simulink model "RoboBoat_SLAM_6_29"  (R2014a)
settings: Solver=FixedStepDiscrete  StartTime=0.0  StopTime=inf  FixedStep=.1  RelTol=1e-3
undefined symbols (not defined in the file): Com1, Com2, Com3, Com4, DiscIntNeverNeededParam, standard
libraries: xpcseriallib x29, visiontextngfix x25, simulink x21, slrtlib x7, speedgoatlib_IO102 x5, speedgoatlib x1
(part 2 of 6)

== matlab function RoboBoat_SLAM_6_29/Main FSM/Obstacle Navigation1/Exit Gate/Gate 1 (Red & White)/MATLAB Function ==
  data: Prob input; RPM output; ColorID input; Dist input; Ang input; CurrentHeading input; GPSLat input; GPSLong input; Timer input; DesiredHeading output; gateGPS output
function [RPM,DesiredHeading,gateGPS] = navigation(Prob,ColorID,Dist,Ang,CurrentHeading,GPSLat,GPSLong,Timer)

% Function performs one buoy navigation through the start speed gates. If
% no buoys are found by the LIDAR/Vision assembly then an incremented
% turning algorithm is executed to turn by 10 degrees per increment up to 
% 90 degrees either way of the inital heading

% Written by Edward Zhu

persistent LockHeading TimeLastFound Counter Turn TurnInc gateLat gateLong

if isempty(LockHeading) && isempty(TimeLastFound) && isempty(Counter) && isempty(Turn) && isempty(TurnInc)
    LockHeading = CurrentHeading;
    TimeLastFound = 0;
    Counter = 0;
    TurnInc = 30;
    Turn = TurnInc;
    gateLat = 0;
    gateLong = 0;
end

Distance = Dist/100;

BoatWidth = 0.75;
Buffer = atan(2*BoatWidth/Distance);

RedOffset = Ang + Buffer;
WhiteOffset = Ang - Buffer;

R = 6378137;

CurLat = (floor(GPSLat/100)+mod(GPSLat,100)/60)*pi/180;
CurLong = (ceil(GPSLong/100)-mod(-GPSLong,100)/60)*pi/180;

gateHeading = (mod(CurrentHeading + Ang, 360))*pi/180;

if ColorID == 1 && Prob > 0.9
    if Ang < 0
        DesiredHeading = mod(CurrentHeading - RedOffset, 360);
    else
        DesiredHeading = mod(CurrentHeading + RedOffset, 360);
    end
    RPM = 4000;
    GateFound = 1;
    TimeLastFound = Timer;
    gateLat =  asin(sin(CurLat)*cos(Distance/R) + cos(CurLat)*sin(Distance/R)*cos(gateHeading))*180/pi;
    gateLong = (CurLong + atan2(sin(gateHeading)*sin(Distance/R)*cos(CurLat),cos(Distance/R)-sin(CurLat)*sin(gateLat)))*180/pi;
elseif ColorID == 2 && Prob > 0.9
    DesiredHeading = mod(LockHeading - Turn, 360);
    RPM = 0;
    GateFound = 1;
    TimeLastFound = Timer;
%     DesiredHeading = mod(CurrentHeading - WhiteOffset, 360);
%     RPM = 4000;
%     GateFound = 1;
%     TimeLastFound = Timer;
%     gateLat =  asin(sin(CurLat)*cos(Distance/R) + cos(CurLat)*sin(Distance/R)*cos(gateHeading))*180/pi;
%     gateLong = (CurLong + atan2(sin(gateHeading)*sin(Distance/R)*cos(CurLat),cos(Distance/R)-sin(CurLat)*sin(gateLat)))*180/pi;
else
    DesiredHeading = CurrentHeading;
    RPM = 0;
    GateFound = 0;
end

gateGPS = [gateLat gateLong];
TimeNoBuoys = Timer - TimeLastFound;

if GateFound == 0 && TimeNoBuoys > 15
    RPM = 0;
    DesiredHeading = mod(LockHeading - Turn, 360);
    HeadingDiff = DesiredHeading - CurrentHeading;
    gateGPS = [gateLat gateLong];
    
    if HeadingDiff > 180
        HeadingDiff = HeadingDiff - 360;
    elseif HeadingDiff < -180
        HeadingDiff = HeadingDiff + 360;
    end
    
    if HeadingDiff < 3
        Counter = Counter + 1;
    else
        Counter = 0;
    end
    
    if Counter >= 15
        Turn = Turn + TurnInc;
        Counter = 0;
        if abs(Turn) > 90
            TurnInc = -TurnInc;
        end
    end
end

== matlab function RoboBoat_SLAM_6_29/Main FSM/Start Speed/GPS Enabler ==
  data: Finished input; SSMode output; Gate1 output; Gate2 output
function [SSMode, Gate1, Gate2] = GPSEnable(Finished)

%Written by Anderson Lebbad on June 9, 2015
%Last Edited: June 10, 2015
%
%This function enables Speedgate tasks. First the searches for and
%navigates through one gate, then the second.

%Initialize Enablers
Gate1 = 0;
Gate2 = 0;


%Switches the enable signal based on which task is flagged as done.
if Finished == 0
    Gate1 = 1;
    SSMode = 1;
else
    Gate2 = 1;
    SSMode = 2;
end

== matlab function RoboBoat_SLAM_6_29/Main FSM/Start Speed/Gate Find and Through/Find/MATLAB Function1 ==
  data: Dist input; Angles input; X input; Y input; Heading input; found output; Goal output; DesiredHeading output
function [found, Goal, DesiredHeading] = SpeedGate(Dist,Angles,X,Y,Heading)
%Written by Anderson Lebbad on May 29, 2015
%Last Edited by:

%This function sends theboat forward until a landmark is found, then it
%navigates towards the right of it.

persistent goalX goalY Found initialHeading change
if isempty(goalX)
    goalX = X;
    goalY = Y;
    Found = 0;
    initialHeading = Heading;
    change = 10;
end

DesiredHeading = Heading;
DistM = Dist./100;
dodgeWidth = 3;

if Found == 0
    if DistM(2) ~= 0
        %If two objects are found, set goal between the two
        w = (DistM(1)*sin(Angles(1)) + DistM(2)*sin(Angles(2)*pi/180)) / 2;
        h = (DistM(1)*cos(Angles(1)) + DistM(2)*sin(Angles(2)*pi/180)) / 2;
        goalX = X + h*cos(Heading) - w*sin(Heading);
        goalY = Y + h*sin(Heading) + w*cos(Heading);
        Found = 1;
    elseif DistM(1) ~= 0
        %If one object is found, set goal dodgewidth to the right of it
        w = DistM(1)*sin(Angles(1)) + dodgeWidth;
        h = DistM(1)*cos(Angles(1));
        goalX = X + h*cos(Heading) - w*sin(Heading);
        goalY = Y + h*sin(Heading) + w*cos(Heading);
        Found = 1;
    else
        %If no objects are found, search. Scan 30 degrees to left and right
        %of initial heading.
        DesiredHeading = Heading + change;
        if abs(DesiredHeading - initialHeading) > 30
            change = -change;
            DesiredHeading = Heading + change;
        end
    end
end

Goal = [goalX, goalY];
found = Found;

end

== matlab function RoboBoat_SLAM_6_29/Main FSM/Obstacle Navigation1/Enter Gate/Gate 2 (White & White)/Distance ==
  data: Distance output; DesiredGPS input; GPSLat input; GPSLong input
function Distance  = DistCalc(DesiredGPS, GPSLat, GPSLong)

%Written by Anderson Lebbad on July 22, 2013
%Last Edited:

%Orients the boat towards a target GPS point before approaching it.
%This is done to keep the approach angle minimal, so the approach
%algorithm does not circle the target and never reach it.

%Parse input GPS and convert angles to radians
CurLat = (floor(GPSLat/100)+mod(GPSLat,100)/60)*pi/180;
CurLong = (floor(GPSLong/100)+mod(GPSLong,100)/60)*pi/180;
DesLat = (floor(DesiredGPS(1)/100)+mod(DesiredGPS(1),100)/60)*pi/180;
DesLong = (floor(DesiredGPS(2)/100)+mod(DesiredGPS(2),100)/60)*pi/180;
%Difference between lats and longs
DiffLat = DesLat - CurLat;
MidLat = cos((CurLat + DesLat)/2);
DiffLong = DesLong - CurLong;
%Radius of the earth in meters
R = 6378137;

%Calculate distance using the great-circle distance formula
%Formula documented here:
%   http://www.movable-type.co.uk/scripts/latlong.html
% a = sin(DiffLat/2)^2+sin(DiffLong/2)^2*cos(CurLat)*cos(DesLat);
% c = 2*atan2(sqrt(a), sqrt(1-a));
% Distance = R*c;

%Calculating distance using Pythagora's
a = DiffLong*MidLat;
b = DiffLat;
Distance = R*sqrt(a^2+b^2);

== matlab function RoboBoat_SLAM_6_29/Main FSM/Obstacle Navigation1/Enter Gate/MATLAB Function ==
  data: gateID input; outputSelector output; gate1En output; gate2En output; gate3En output
function [outputSelector,gate1En,gate2En,gate3En] = gateSelector(gateID)
% Determines which colors to filter for based on the gateID as received
% from the judges

gate1En = 0;
gate2En = 0;
gate3En = 0;

if gateID == 1
    gate1En = 1;
    outputSelector = 1;
elseif gateID == 2
    gate2En = 1;
    outputSelector = 2;
else
    gate3En = 1;
    outputSelector = 3;
end

== matlab function RoboBoat_SLAM_6_29/Main FSM/Obstacle Navigation1/Obstacle Navigation/GPS: Bee Line/Orient/Desired Heading ==
  data: DesiredGPS input; DesiredHeading output; GPSLat input; GPSLong input
function DesiredHeading = Orient(DesiredGPS, GPSLat, GPSLong)

%Written by Anderson Lebbad on July 22, 2013
%Last Edited: Edward Zhu on July 5, 2014

% Edit:
% Changed calculation to use positive lat and negative long

%Orients the boat towards a target GPS point before approaching it.
%This is done to keep the approach angle minimal, so the approach
%algorithm does not circle the target and never reach it.

%Parse input GPS and convert angles to radians
CurLat = (floor(GPSLat/100)+mod(GPSLat,100)/60)*pi/180;
CurLong = (ceil(GPSLong/100)-mod(-GPSLong,100)/60)*pi/180;
DesLat = (floor(DesiredGPS(1)/100)+mod(DesiredGPS(1),100)/60)*pi/180;
DesLong = (ceil(DesiredGPS(2)/100)-mod(-DesiredGPS(2),100)/60)*pi/180;

%Difference between longs
DiffLong = DesLong - CurLong;

%Calculate initial bearing - formula documented here: 
%   http://www.movable-type.co.uk/scripts/latlong.html
y = sin(DiffLong)*cos(DesLat);
x = cos(CurLat)*sin(DesLat)-sin(CurLat)*cos(DesLat)*cos(DiffLong);
DesiredHeading = mod(atan2(y, x)*180/pi + 360, 360);

== matlab function RoboBoat_SLAM_6_29/Main FSM/Obstacle Navigation1/GPS: Center/Approach/MATLAB Function ==
  data: GPSLat input; out output; GPSLong input; IMULat input; IMULong input
function out = dataFormat(GPSLat, GPSLong, IMULat, IMULong)
%#codegen
out = [GPSLat GPSLong IMULat IMULong];

== matlab function RoboBoat_SLAM_6_29/Main FSM/Obstacle Navigation1/GPS: Center/Orient/Desired Heading ==
  data: DesiredGPS input; DesiredHeading output; GPSLat input; GPSLong input
function DesiredHeading = Orient(DesiredGPS, GPSLat, GPSLong)

%Written by Anderson Lebbad on July 22, 2013
%Last Edited: Edward Zhu on July 5, 2014

% Edit:
% Changed calculation to use positive lat and negative long

%Orients the boat towards a target GPS point before approaching it.
%This is done to keep the approach angle minimal, so the approach
%algorithm does not circle the target and never reach it.

%Parse input GPS and convert angles to radians
CurLat = (floor(GPSLat/100)+mod(GPSLat,100)/60)*pi/180;
CurLong = (ceil(GPSLong/100)-mod(-GPSLong,100)/60)*pi/180;
DesLat = (floor(DesiredGPS(1)/100)+mod(DesiredGPS(1),100)/60)*pi/180;
DesLong = (ceil(DesiredGPS(2)/100)-mod(-DesiredGPS(2),100)/60)*pi/180;

%Difference between longs
DiffLong = DesLong - CurLong;

%Calculate initial bearing - formula documented here: 
%   http://www.movable-type.co.uk/scripts/latlong.html
y = sin(DiffLong)*cos(DesLat);
x = cos(CurLat)*sin(DesLat)-sin(CurLat)*cos(DesLat)*cos(DiffLong);
DesiredHeading = mod(atan2(y, x)*180/pi + 360, 360);

== matlab function RoboBoat_SLAM_6_29/Main FSM/Obstacle Navigation1/Obstacle Navigation/GPS: Bee Line/Approach/Desired Heading and Distance ==
  data: Distance output; DesiredGPS input; DesiredHeading output; GPSLat input; GPSLong input
function [Distance, DesiredHeading] = Approach(DesiredGPS, GPSLat, GPSLong)

%Written by Anderson Lebbad on July 22, 2013
%Last Edited: Edward Zhu July 5, 2014

%Edit:
% Switched from great-circle distance formula to equirectangular approx and
%used mod for desired heading
% Changed calculation to use positve lat and negative long

%Orients the boat towards a target GPS point before approaching it.
%This is done to keep the approach angle minimal, so the approach
%algorithm does not circle the target and never reach it.

%Parse input GPS and convert angles to radians
CurLat = (floor(GPSLat/100)+mod(GPSLat,100)/60)*pi/180;
CurLong = (ceil(GPSLong/100)-mod(-GPSLong,100)/60)*pi/180;
DesLat = (floor(DesiredGPS(1)/100)+mod(DesiredGPS(1),100)/60)*pi/180;
DesLong = (ceil(DesiredGPS(2)/100)-mod(-DesiredGPS(2),100)/60)*pi/180;

%Difference between lats and longs
DiffLat = DesLat - CurLat;
MidLat = cos((CurLat + DesLat)/2);
DiffLong = DesLong - CurLong;

%Radius of the earth in meters
R = 6378137;

%Calculate distance using the great-circle distance formula
%Formula documented here:
%   http://www.movable-type.co.uk/scripts/latlong.html
% a = sin(DiffLat/2)^2+sin(DiffLong/2)^2*cos(CurLat)*cos(DesLat);
% c = 2*atan2(sqrt(a), sqrt(1-a));
% Distance = R*c;

%Calculating distance using equirectangular approximation since distances
%concerned are very small
a = DiffLong*MidLat;
b = DiffLat;
Distance = R*sqrt(a^2+b^2);

%Calculate initial bearing - formula documented here: 
%   http://www.movable-type.co.uk/scripts/latlong.html
y = sin(DiffLong)*cos(DesLat);
x = cos(CurLat)*sin(DesLat)-sin(CurLat)*cos(DesLat)*cos(DiffLong);
DesiredHeading = mod(atan2(y, x)*180/pi + 360, 360);

== matlab function RoboBoat_SLAM_6_29/Sensors/1020 Comms/MATLAB Function2 ==
  data: Time input; asciiLIT output; Sequence input
% This function creates the light tower message to be sent from 
% Speedgoat in ascii code
% Written by: Edward Zhu
% Date: 9/17/14

function asciiLIT = asciiLITEncoder(Time, Sequence)

% Initialize output message vector as the serial output block expects 128
% character message
asciiLIT = uint8(zeros(1,128));

% Convert static strings to ascii code
asciiMsgID = uint8('$RXLIT,');
asciiComma = uint8(',');
asciiTeamID = uint8('FAUVU,');
asciiMsgEnd = uint8('*');
asciiMsgCRLF = [13 10];

% Convert UTC Time input (hhmmss) into ascii code
asciiTime = uint8(zeros(1,7));
asciiTime(7) = asciiComma;

for timeChar = 1:6
    asciiTime(timeChar) = floor(mod(Time,10^(7-timeChar))/...
        10^(6-timeChar)) + 48;
end

% Convert the light sequece into ascii code (1 = R, 2 = B, 3 = G)
asciiSeq = uint8(zeros(1,4)+32);
asciiSeq(4) = asciiMsgEnd;

if Sequence(1) > 0 && Sequence(2) > 0 && Sequence(3) > 0
    for seqChar = 1:3
        if Sequence(seqChar) == 1
            Sequence(seqChar) = uint8('R');
        elseif Sequence(seqChar) == 2
            Sequence(seqChar) = uint8('B');
        elseif Sequence(seqChar) == 3
            Sequence(seqChar) = uint8('G');
        end
    end
    asciiSeq(1:3) = Sequence;
end

% Concat individual ascii arrays into one array
asciiPreChkSum = cat(2,asciiMsgID,asciiTime,asciiTeamID,asciiSeq);

% Calculate the checksum of the message from the '$' to the '*' and convert
% to hex
chkSum = uint8(0);

for chksumChar = 1:(length(asciiPreChkSum)-2)
    chkSum = bitxor(chkSum,asciiPreChkSum(chksumChar+1));
end

% Convert the checksum to ascii
chkSum = dec2hex(chkSum);
asciiChkSum = uint8(zeros(1,length(chkSum))+32);
for i = 1:length(chkSum)
    asciiChkSum(i) = uint8(chkSum(i));
end

% Concat the checksum and the '/r/n' to the end of the message
asciiPostChkSum = cat(2,asciiPreChkSum,asciiChkSum,asciiMsgCRLF);

% Output the final message
asciiLIT(1:length(asciiPostChkSum)) = asciiPostChkSum;

== matlab function RoboBoat_SLAM_6_29/Main FSM/SLAM/Landmark Organizer ==
  data: Distances input; lm_data output; Angles input
function lm_data = lmOrganize(Distances,Angles)
%Written By Anderson Lebbad on September 16, 2014
%Last Edited by:

%This function structures the landmark data to be used for the SLAM

landmarks = [Distances'; Angles'];
[M,N] = size(landmarks);
lm_data = landmarks(1:M*N);

end

== matlab function RoboBoat_SLAM_6_29/Main FSM/SLAM/SLAM enabled/SLAM RT ==
  data: particle_pose input; pose input; lm_data input; Map output
function Map   = SLAMrt( particle_pose, pose, lm_data )
%Written By Anderson Lebbad on 3/11/2015
%Last Edited by:
%
%
%Implementation of the particular modificaiton of the FastSLAM algorithm
%developed by Nicholas Dileo for real-time application.

%partice_pose - 50 by 3, each particle is a row, with columns of X,Y,Psi
%pose - position of the boat in NED, X,Y,Psi
%lm_data - 12 by 2. Rows are identified targets, columns are [d,theta]

%% Initialization

%Field of view parameters
max_read_distance = 10;
min_read_distance = 5;
max_read_angle = 67*pi/180;
min_read_angle = -67*pi/180;


%max_num_lm - Sets the absolute maximum number of landmarks that a
%particle can track
max_num_lm = 50;

%intialize output
Map = nan(max_num_lm,2);

%num_particles - Defines the number of particles for the particle filter.
%Needs to match the number of models running outside the function
num_particles = 50;

%Landmark matrix - Tracks distances and angles for the landmarks detected
%by each particle
persistent landmarks;
if isempty(landmarks)
    landmarks = nan(max_num_lm,2,num_particles);
end
%count matrix - Keeps track of how many times a landmark has been detected,
%minus the amount of times the landmark failed to be detected in view for
%the first column. The second column tracks how recently the landmark was
%detected, so older landmarks get pushed out if maximum number of landmarks
%has been reached.
persistent count;
if isempty(count)
    count = zeros(max_num_lm,2,num_particles);
end
%newly detected landmarks converted into NED coordinates
lm_NED = [pose(1)+lm_data(:,1).*cos(pose(3)+lm_data(:,2)), ...
    pose(2)+lm_data(:,1).*sin(pose(3)+lm_data(:,2))];
%wherever the distance is equal to 0 is invalid
new_lm_valids = lm_data(:,1) ~= 0;
%invalids are NaN
lm_NED(~new_lm_valids,:) = NaN;
%Variable for holding all landmark data together in one list, for
%generating output map
all_lms = nan(max_num_lm*num_particles,2);

%% Loop through each particle

for pIdx = 1:num_particles
    %% Cluster new data with old
    
    %Check how many landmarks have been tracked for this particle
    old_lm_valids = ~isnan(landmarks(:,1,pIdx));
    %Create an evaluation matrix to cluster the new detections with
    %previously identified landmarks
    evalMat = [landmarks(:,:,pIdx); lm_NED];
    %clustering together
    [Inds, Means] = clusterRT(evalMat, 0.3);
    %split the index matrix for the clusters between new data and old to
    %see if landmarks need to be removed from the current list to make room
    %for new data
    newInds = Inds(max_num_lm+1:max_num_lm+length(new_lm_valids));
    oldInds = Inds(1:max_num_lm);
    
    %% Increment count variable, and evaluate if landmarks should be removed
    
    %find which old landmarks should be detected this frame
    old_lm_dist = sqrt((landmarks(:,1,pIdx)-particle_pose(pIdx,1)).^2 + ...
        (landmarks(:,2,pIdx)-particle_pose(pIdx,2)).^2);
    old_lm_angle = atan2(landmarks(:,2,pIdx)-particle_pose(pIdx,2),...
        landmarks(:,1,pIdx)-particle_pose(pIdx,1)) - particle_pose(pIdx,3);
    rmax = max_read_distance*ones(max_num_lm,1);
    rmin = min_read_distance*ones(max_num_lm,1);
    amax = max_read_angle*ones(max_num_lm,1);
    amin = min_read_angle*ones(max_num_lm,1);
    rbmax = old_lm_dist < rmax;
    ramin = old_lm_dist > rmin;
    abmax = old_lm_angle < amax;
    aamin = old_lm_angle > amin;
    lm_in_frame = rbmax.*ramin.*abmax.*aamin;
    %increment last seen column of count (anything recently seen will be
    %cleared later)
    count(:,2,pIdx) = count(:,2,pIdx) + 1;
    %update the seen unseen column of count
    [B,I] = sort(newInds(new_lm_valids));
    [seen, J] = ismember(oldInds.*lm_in_frame,B);
    where_seen = I(J(seen));
    unseen = logical(lm_in_frame - seen);
    count(seen,1,pIdx) = count(seen,1,pIdx) + 1;
    count(unseen,1,pIdx) = count(unseen,1,pIdx) - 1;
    %if count is negative, it has been missed more than it has been seen
    %when it should be in the field of view. Therefore, remove the landmark
    %from the list (or rather, replace with NaNs)
    neg_count = count(:,1,pIdx) < 0;
    Means(oldInds(neg_count),:) = NaN;
    %figure out which old landmarks are still valid, and not updated by
    %new data
    old_lm_valids = old_lm_valids - neg_count - seen;
    %set the last seen column of count to NaN for anything invalid
    count(~old_lm_valids,2,pIdx) = NaN;
    
    %% Update landmarks to new means
    
    %clear old ones off the list
    landmarks(:,:,pIdx) = NaN;
    %the total number of new valid landmarks
    num_new_valids = sum(new_lm_valids);
    %first fill in recently detected landmarks
    landmarks(1:num_new_valids,:,pIdx) = Means(newInds(new_lm_valids),:);
    %sort old landmarks based on recent last seen count
    [~,most_to_least_recent] = sort(count(:,2,pIdx));
    %find how many of the old landmarks should be added to the updated list
    num_updates = min(sum(old_lm_valids),max_num_lm - sum(new_lm_valids));
    %add them to the landmarks list
    landmarks(num_new_valids+1:num_new_valids+num_updates,:,pIdx) = ...
        Means(oldInds(most_to_least_recent(1:num_updates)),:);
    
    %% Update count matrix
    
    %Initialize an update matrix
    new_count = ones(max_num_lm,2);
    %pass the counts for the new readings that have been clustered with
    %previous data (but not the last seen, as that is reset to 1)
    new_count(where_seen,1) = count(seen,1,pIdx);
    %pass the count information for the old clusters
    new_count(num_new_valids+1:num_new_valids+num_updates,:) = ...
        count(most_to_least_recent(1:num_updates),:,pIdx);
    %update counts
    count(:,:,pIdx) = new_count;
    
    %% Add to all landmark list
    
    all_lms((pIdx-1)*max_num_lm+1:pIdx*max_num_lm,:) = landmarks(:,:,pIdx);
end

%% Deal with data association over all particles and output map

%cluster all landmarks
[a_inds, a_means] = clusterRT(all_lms, 0.3);
%find unique values
uniques = unique(a_inds);
%number of occurances of each unique element
occurances = histc(a_inds(~isnan(all_lms(:,1))),uniques);
%sort uniques from max number of occurances
[~,uniqSorted] = sort(occurances,'descend');

num_to_list = min(max_num_lm,sum(occurances > 1));
%include the clustered output, in order of most recognized
Map(1:num_to_list,:) = a_means(uniqSorted(1:num_to_list,1),:);

end

function [ clusterInds, meanVals ] = clusterRT( data, Ssensitivity )
%Written by Anderson Lebbad on 3/11/2015
%Last Edited:
%
%
%Implementation of clustering for real-time operation. Each row is a unique
%data set, with column-wise charateristics. This function groups together
%data sets (row-wise) by those that have been grouped together over all
%columns the same. Tracks means of values for each cluster as well.

[m,n] = size(data);

cClusterInds = zeros(m,n);


sensitivity = Ssensitivity*ones(1,n);


for i = 1:n
    cClusterInds(:,i) = clusterVector(data(:,i),sensitivity(i));
end

% Columnwise clustering is now done. Each element is a member of exactly
% one cluster per column. cClustersInds is a matrix of which column
% cluster each element belongs to. We now cluster across the rows by
% aggregating each set of unique row-wise cluster indices into a unique
% global cluster
[~, ~, clusterInds] = unique(cClusterInds,'rows');

meanVals = nan(m,n);

for j = 1:max(clusterInds)
    meanVals(j,:) = mean(data((clusterInds==j),:),1);
end

end

function [colClusterInds] = clusterVector(vector,coarseness)
%Operates a vector of data, separating by distance between elements
vector= vector(:);
[b,inds] = sort(vector);
diffs = diff([-inf;b]);

maxDiff = max(diffs(isfinite(diffs)));
minDiff = coarseness * maxDiff;

startInds = find(diffs > minDiff);
if numel(startInds) > 1
    endInds = startInds-1;
    endInds = [endInds(2:end);numel(b)];
else
    endInds = numel(b);
end

%Preallocation
colClusterInds = zeros(size(vector));

for ind = 1:numel(startInds)
    colClusterInds(inds(startInds(ind):endInds(ind))) = ind;
end

end

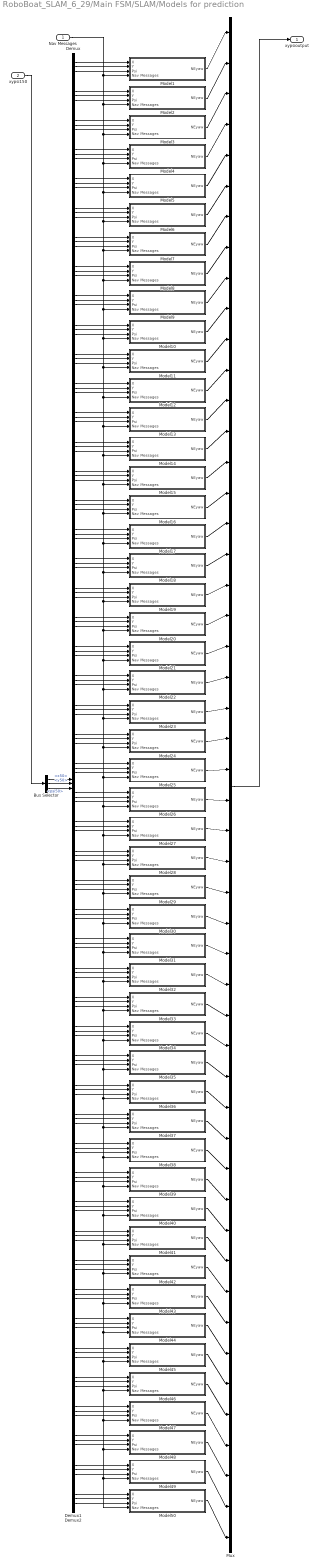
== system RoboBoat_SLAM_6_29/Main FSM/SLAM/Models for prediction ==
  Nav Messages : Inport
  xypsi150 : Inport  Port=2
  Bus Selector : BusSelector  OutputSignals=x50,y50,psi50
  Demux : Demux  Outputs=50
  Demux1 : Demux  Outputs=50
  Demux2 : Demux  Outputs=50
  Model1 : Subsystem
  Model10 : Subsystem
  Model11 : Subsystem
  Model12 : Subsystem
  Model13 : Subsystem
  Model14 : Subsystem
  Model15 : Subsystem
  Model16 : Subsystem
  Model17 : Subsystem
  Model18 : Subsystem
  Model19 : Subsystem
  Model2 : Subsystem
  Model20 : Subsystem
  Model21 : Subsystem
  Model22 : Subsystem
  Model23 : Subsystem
  Model24 : Subsystem
  Model25 : Subsystem
  Model26 : Subsystem
  Model27 : Subsystem
  Model28 : Subsystem
  Model29 : Subsystem
  Model3 : Subsystem
  Model30 : Subsystem
  Model31 : Subsystem
  Model32 : Subsystem
  Model33 : Subsystem
  Model34 : Subsystem
  Model35 : Subsystem
  Model36 : Subsystem
  Model37 : Subsystem
  Model38 : Subsystem
  Model39 : Subsystem
  Model4 : Subsystem
  Model40 : Subsystem
  Model41 : Subsystem
  Model42 : Subsystem
  Model43 : Subsystem
  Model44 : Subsystem
  Model45 : Subsystem
  Model46 : Subsystem
  Model47 : Subsystem
  Model48 : Subsystem
  Model49 : Subsystem
  Model5 : Subsystem
  Model50 : Subsystem
  Model6 : Subsystem
  Model7 : Subsystem
  Model8 : Subsystem
  Model9 : Subsystem
  Mux : Mux  Inputs=50
  xypsioutput : Outport  PortDimensions=150
  wires:
  Demux/1 -> Model1/1(X)
  Demux1/1 -> Model1/2(Y)
  Demux2/1 -> Model1/3(Psi)
  Demux/2 -> Model2/1(X)
  Demux1/2 -> Model2/2(Y)
  Demux2/2 -> Model2/3(Psi)
  Demux/3 -> Model3/1(X)
  Demux1/3 -> Model3/2(Y)
  Demux2/3 -> Model3/3(Psi)
  Demux/4 -> Model4/1(X)
  Demux1/4 -> Model4/2(Y)
  Demux2/4 -> Model4/3(Psi)
  Demux/5 -> Model5/1(X)
  Demux1/5 -> Model5/2(Y)
  Demux2/5 -> Model5/3(Psi)
  Demux/6 -> Model6/1(X)
  Demux1/6 -> Model6/2(Y)
  Demux2/6 -> Model6/3(Psi)
  Nav Messages/1 -> Model2/4(Nav Messages), Model3/4(Nav Messages), Model4/4(Nav Messages), Model5/4(Nav Messages), Model6/4(Nav Messages), Model7/4(Nav Messages), Model8/4(Nav Messages), Model9/4(Nav Messages), Model10/4(Nav Messages), Model11/4(Nav Messages), Model12/4(Nav Messages), Model13/4(Nav Messages), Model14/4(Nav Messages), Model15/4(Nav Messages), Model16/4(Nav Messages), Model17/4(Nav Messages), Model18/4(Nav Messages), Model19/4(Nav Messages), Model20/4(Nav Messages), Model21/4(Nav Messages), Model22/4(Nav Messages), Model23/4(Nav Messages), Model24/4(Nav Messages), Model25/4(Nav Messages), Model26/4(Nav Messages), Model27/4(Nav Messages), Model28/4(Nav Messages), Model29/4(Nav Messages), Model30/4(Nav Messages), Model31/4(Nav Messages), Model32/4(Nav Messages), Model33/4(Nav Messages), Model34/4(Nav Messages), Model35/4(Nav Messages), Model36/4(Nav Messages), Model37/4(Nav Messages), Model38/4(Nav Messages), Model39/4(Nav Messages), Model40/4(Nav Messages), Model41/4(Nav Messages), Model42/4(Nav Messages), Model43/4(Nav Messages), Model44/4(Nav Messages), Model45/4(Nav Messages), Model46/4(Nav Messages), Model47/4(Nav Messages), Model48/4(Nav Messages), Model50/4(Nav Messages), Model49/4(Nav Messages), Model1/4(Nav Messages)
  Demux2/15 -> Model15/3(Psi)
  Demux1/15 -> Model15/2(Y)
  Demux/15 -> Model15/1(X)
  Demux2/14 -> Model14/3(Psi)
  Demux1/14 -> Model14/2(Y)
  Demux/14 -> Model14/1(X)
  Demux2/13 -> Model13/3(Psi)
  Demux1/13 -> Model13/2(Y)
  Demux/13 -> Model13/1(X)
  Demux2/12 -> Model12/3(Psi)
  Demux1/12 -> Model12/2(Y)
  Demux/12 -> Model12/1(X)
  Demux2/11 -> Model11/3(Psi)
  Demux1/11 -> Model11/2(Y)
  Demux/11 -> Model11/1(X)
  Demux2/10 -> Model10/3(Psi)
  Demux1/10 -> Model10/2(Y)
  Demux/10 -> Model10/1(X)
  Demux2/9 -> Model9/3(Psi)
  Demux1/9 -> Model9/2(Y)
  Demux/9 -> Model9/1(X)
  Demux2/8 -> Model8/3(Psi)
  Demux1/8 -> Model8/2(Y)
  Demux/8 -> Model8/1(X)
  Demux2/7 -> Model7/3(Psi)
  Demux1/7 -> Model7/2(Y)
  Demux/7 -> Model7/1(X)
  Demux/16 -> Model16/1(X)
  Demux1/16 -> Model16/2(Y)
  Demux2/16 -> Model16/3(Psi)
  Demux/17 -> Model17/1(X)
  Demux1/17 -> Model17/2(Y)
  Demux2/17 -> Model17/3(Psi)
  Demux/18 -> Model18/1(X)
  Demux1/18 -> Model18/2(Y)
  Demux2/18 -> Model18/3(Psi)
  Demux/19 -> Model19/1(X)
  Demux1/19 -> Model19/2(Y)
  Demux2/19 -> Model19/3(Psi)
  Demux/20 -> Model20/1(X)
  Demux1/20 -> Model20/2(Y)
  Demux2/20 -> Model20/3(Psi)
  Demux/21 -> Model21/1(X)
  Demux1/21 -> Model21/2(Y)
  Demux2/21 -> Model21/3(Psi)
  Demux/22 -> Model22/1(X)
  Demux1/22 -> Model22/2(Y)
  Demux2/22 -> Model22/3(Psi)
  Demux/23 -> Model23/1(X)
  Demux1/23 -> Model23/2(Y)
  Demux2/23 -> Model23/3(Psi)
  Demux/24 -> Model24/1(X)
  Demux1/24 -> Model24/2(Y)
  Demux2/24 -> Model24/3(Psi)
  Demux/25 -> Model25/1(X)
  Demux1/25 -> Model25/2(Y)
  Demux2/25 -> Model25/3(Psi)
  Demux/26 -> Model26/1(X)
  Demux1/26 -> Model26/2(Y)
  Demux2/26 -> Model26/3(Psi)
  Demux/27 -> Model27/1(X)
  Demux1/27 -> Model27/2(Y)
  Demux2/27 -> Model27/3(Psi)
  Demux/28 -> Model28/1(X)
  Demux1/28 -> Model28/2(Y)
  Demux2/28 -> Model28/3(Psi)
  Demux/29 -> Model29/1(X)
  Demux1/29 -> Model29/2(Y)
  Demux2/29 -> Model29/3(Psi)
  Demux/30 -> Model30/1(X)
  Demux1/30 -> Model30/2(Y)
  Demux2/30 -> Model30/3(Psi)
  Demux/31 -> Model31/1(X)
  Demux1/31 -> Model31/2(Y)
  Demux2/31 -> Model31/3(Psi)
  Demux/32 -> Model32/1(X)
  Demux1/32 -> Model32/2(Y)
  Demux2/32 -> Model32/3(Psi)
  Demux/33 -> Model33/1(X)
  Demux1/33 -> Model33/2(Y)
  Demux2/33 -> Model33/3(Psi)
  Demux/34 -> Model34/1(X)
  Demux1/34 -> Model34/2(Y)
  Demux2/34 -> Model34/3(Psi)
  Demux/35 -> Model35/1(X)
  Demux1/35 -> Model35/2(Y)
  Demux2/35 -> Model35/3(Psi)
  Demux/36 -> Model36/1(X)
  Demux1/36 -> Model36/2(Y)
  Demux2/36 -> Model36/3(Psi)
  Demux/37 -> Model37/1(X)
  Demux1/37 -> Model37/2(Y)
  Demux2/37 -> Model37/3(Psi)
  Demux/38 -> Model38/1(X)
  Demux1/38 -> Model38/2(Y)
  Demux2/38 -> Model38/3(Psi)
  Demux/39 -> Model39/1(X)
  Demux1/39 -> Model39/2(Y)
  Demux2/39 -> Model39/3(Psi)
  Demux/40 -> Model40/1(X)
  Demux1/40 -> Model40/2(Y)
  Demux2/40 -> Model40/3(Psi)
  Demux/41 -> Model41/1(X)
  Demux1/41 -> Model41/2(Y)
  Demux2/41 -> Model41/3(Psi)
  Demux/42 -> Model42/1(X)
  Demux1/42 -> Model42/2(Y)
  Demux2/42 -> Model42/3(Psi)
  Demux/43 -> Model43/1(X)
  Demux1/43 -> Model43/2(Y)
  Demux2/43 -> Model43/3(Psi)
  Demux/44 -> Model44/1(X)
  Demux1/44 -> Model44/2(Y)
  Demux2/44 -> Model44/3(Psi)
  Demux/45 -> Model45/1(X)
  Demux1/45 -> Model45/2(Y)
  Demux2/45 -> Model45/3(Psi)
  Demux/46 -> Model46/1(X)
  Demux1/46 -> Model46/2(Y)
  Demux2/46 -> Model46/3(Psi)
  Demux/47 -> Model47/1(X)
  Demux1/47 -> Model47/2(Y)
  Demux2/47 -> Model47/3(Psi)
  Demux/48 -> Model48/1(X)
  Demux1/48 -> Model48/2(Y)
  Demux2/48 -> Model48/3(Psi)
  Demux/49 -> Model49/1(X)
  Demux1/49 -> Model49/2(Y)
  Demux2/49 -> Model49/3(Psi)
  Demux/50 -> Model50/1(X)
  Demux1/50 -> Model50/2(Y)
  Demux2/50 -> Model50/3(Psi)
  xypsi150/1 -> Bus Selector/1
  Bus Selector/1 -> Demux/1  "<x50>"
  Bus Selector/2 -> Demux1/1  "<y50>"
  Bus Selector/3 -> Demux2/1  "<psi50>"
  Model27/1(NEyaw) -> Mux/27
  Model26/1(NEyaw) -> Mux/26
  Model25/1(NEyaw) -> Mux/25
  Model24/1(NEyaw) -> Mux/24
  Model28/1(NEyaw) -> Mux/28
  Model23/1(NEyaw) -> Mux/23
  Model21/1(NEyaw) -> Mux/21
  Model30/1(NEyaw) -> Mux/30
  Model29/1(NEyaw) -> Mux/29
  Model22/1(NEyaw) -> Mux/22
  Model40/1(NEyaw) -> Mux/40
  Model33/1(NEyaw) -> Mux/33
  Model36/1(NEyaw) -> Mux/36
  Model38/1(NEyaw) -> Mux/38
  Model37/1(NEyaw) -> Mux/37
  Model35/1(NEyaw) -> Mux/35
  Model39/1(NEyaw) -> Mux/39
  Model31/1(NEyaw) -> Mux/31
  Model32/1(NEyaw) -> Mux/32
  Model34/1(NEyaw) -> Mux/34
  Model2/1(NEyaw) -> Mux/2
  Model5/1(NEyaw) -> Mux/5
  Model3/1(NEyaw) -> Mux/3
  Model4/1(NEyaw) -> Mux/4
  Model19/1(NEyaw) -> Mux/19
  Model13/1(NEyaw) -> Mux/13
  Model14/1(NEyaw) -> Mux/14
  Model12/1(NEyaw) -> Mux/12
  Model16/1(NEyaw) -> Mux/16
  Model17/1(NEyaw) -> Mux/17
  Model18/1(NEyaw) -> Mux/18
  Model20/1(NEyaw) -> Mux/20
  Model11/1(NEyaw) -> Mux/11
  Model15/1(NEyaw) -> Mux/15
  Model10/1(NEyaw) -> Mux/10
  Model8/1(NEyaw) -> Mux/8
  Model9/1(NEyaw) -> Mux/9
  Model7/1(NEyaw) -> Mux/7
  Model6/1(NEyaw) -> Mux/6
  Model48/1(NEyaw) -> Mux/48
  Model42/1(NEyaw) -> Mux/42
  Model49/1(NEyaw) -> Mux/49
  Model47/1(NEyaw) -> Mux/47
  Model50/1(NEyaw) -> Mux/50
  Model43/1(NEyaw) -> Mux/43
  Model45/1(NEyaw) -> Mux/45
  Model44/1(NEyaw) -> Mux/44
  Model46/1(NEyaw) -> Mux/46
  Model41/1(NEyaw) -> Mux/41
  Model1/1(NEyaw) -> Mux/1
  Mux/1 -> xypsioutput/1

== system RoboBoat_SLAM_6_29/Main FSM/SLAM/SLAM enabled ==
  pre_past_positions : Inport
  lm_data : Inport  Port=2
  pose : Inport  Port=3
  Enable : EnablePort
  Part Pos : MATLAB Function  TreatAsAtomicUnit=on
  SLAM RT : MATLAB Function  TreatAsAtomicUnit=on
  dataMat : MATLAB Function  TreatAsAtomicUnit=on
  mpa : Outport
  part_positions : Outport  Port=2
  wires:
  lm_data/1 -> dataMat/1(lm_data)
  pre_past_positions/1 -> Part Pos/1(part_positions), part_positions/1
  SLAM RT/1(Map) -> mpa/1
  pose/1 -> SLAM RT/2(pose)
  Part Pos/1(particle_pose) -> SLAM RT/1(particle_pose)
  dataMat/1(lm_data_mat) -> SLAM RT/3(lm_data)

== system RoboBoat_SLAM_6_29/Main FSM/SLAM/inputselection ==
  controlchange : Inport
  xypsi : Inport  Port=2
  Landmarkchange : Inport  Port=3
  part_positions : Inport  Port=4
  xypsi150 : Inport  Port=5
  Bus Creator : BusCreator  Inputs=3
  Delay{,1..4} (5 alike) : Delay  DelayLength=1  InitialCondition=0
  MATLAB Function : MATLAB Function  TreatAsAtomicUnit=on
  last particle positions : Outport
  wires:
  Delay/1 -> MATLAB Function/4(part_positions)
  Delay1/1 -> MATLAB Function/3(xypsi)
  Delay2/1 -> MATLAB Function/5(xypsi150)
  Delay4/1 -> MATLAB Function/1(Landmarkchange)
  Delay3/1 -> MATLAB Function/2(controlchange)
  controlchange/1 -> Delay3/1
  xypsi/1 -> Delay1/1
  part_positions/1 -> Delay/1
  Landmarkchange/1 -> Delay4/1
  xypsi150/1 -> Delay2/1
  MATLAB Function/2(y50) -> Bus Creator/2  "y50"
  MATLAB Function/3(psi50) -> Bus Creator/3  "psi50"
  MATLAB Function/1(x50) -> Bus Creator/1  "x50"
  Bus Creator/1 -> last particle positions/1  "last particle positions"

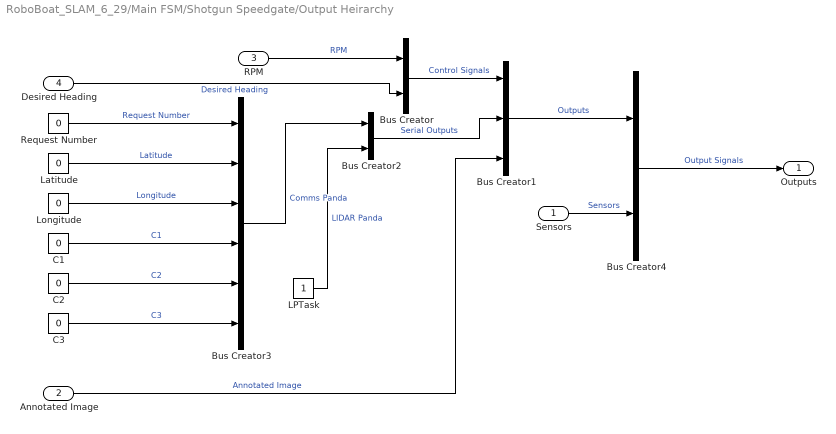
== system RoboBoat_SLAM_6_29/Main FSM/Shotgun Speedgate/Output Heirarchy ==
  Sensors : Inport
  Annotated Image : Inport  Port=2
  RPM : Inport  Port=3
  Desired Heading : Inport  Port=4
  Bus Creator : BusCreator  Inputs=2
  Bus Creator1 : BusCreator  Inputs=3
  Bus Creator2 : BusCreator  Inputs=2
  Bus Creator3 : BusCreator  Inputs=6
  Bus Creator4 : BusCreator  Inputs=2
  C1 : Constant  Value=0
  C2 : Constant  Value=0
  C3 : Constant  Value=0
  LPTask : Constant
  Latitude : Constant  Value=0
  Longitude : Constant  Value=0
  Request Number : Constant  Value=0
  Outputs : Outport
  wires:
  Bus Creator/1 -> Bus Creator1/1  "Control Signals"
  Bus Creator3/1 -> Bus Creator2/1  "Comms Panda"
  Request Number/1 -> Bus Creator3/1  "Request Number"
  Latitude/1 -> Bus Creator3/2  "Latitude"
  Longitude/1 -> Bus Creator3/3  "Longitude"
  C1/1 -> Bus Creator3/4  "C1"
  LPTask/1 -> Bus Creator2/2  "LIDAR Panda"
  Bus Creator1/1 -> Bus Creator4/1  "Outputs"
  Annotated Image/1 -> Bus Creator1/3  "Annotated Image"
  Sensors/1 -> Bus Creator4/2  "Sensors"
  Bus Creator4/1 -> Outputs/1  "Output Signals"
  Bus Creator2/1 -> Bus Creator1/2  "Serial Outputs"
  C2/1 -> Bus Creator3/5  "C2"
  C3/1 -> Bus Creator3/6  "C3"
  RPM/1 -> Bus Creator/1  "RPM"
  Desired Heading/1 -> Bus Creator/2  "Desired Heading"

== system RoboBoat_SLAM_6_29/Main FSM/Start Speed/Gate Find and Through ==
  Sensors : Inport
  Enable : EnablePort
  Find : Subsystem  TreatAsAtomicUnit=on
  GPS Enabler : MATLAB Function  TreatAsAtomicUnit=on
  GPS Selector : MultiPortSwitch  Inputs=2
  Through : Subsystem  TreatAsAtomicUnit=on
  Unit Delay : UnitDelay  SampleTime=-1
  Unit Delay1 : UnitDelay  SampleTime=-1
  Outputs : Outport
  Finished : Outport  Port=2
  wires:
  Sensors/1 -> Through/1(Sensors), Find/1(Sensors)
  GPS Enabler/2(OrientEn) -> Find/Enable
  GPS Enabler/3(ApproachEn) -> Through/Enable
  Find/2(Finished) -> Unit Delay/1
  Find/1(Outputs) -> GPS Selector/2
  Through/1(Outputs) -> GPS Selector/3
  GPS Enabler/1(GPSMode) -> GPS Selector/1
  Unit Delay/1 -> GPS Enabler/1(Finished)
  GPS Selector/1 -> Outputs/1
  Through/2(Finished) -> Unit Delay1/1
  Unit Delay1/1 -> Finished/1

== system RoboBoat_SLAM_6_29/Main FSM/Start Speed/Gate Find and Through1 ==
  Sensors : Inport
  Enable : EnablePort
  Find : Subsystem  TreatAsAtomicUnit=on
  GPS Enabler : MATLAB Function  TreatAsAtomicUnit=on
  GPS Selector : MultiPortSwitch  Inputs=2
  Through : Subsystem  TreatAsAtomicUnit=on
  Unit Delay : UnitDelay  SampleTime=-1
  Unit Delay1 : UnitDelay  SampleTime=-1
  Outputs : Outport
  Finished : Outport  Port=2
  wires:
  Sensors/1 -> Through/1(Sensors), Find/1(Sensors)
  GPS Enabler/2(OrientEn) -> Find/Enable
  GPS Enabler/3(ApproachEn) -> Through/Enable
  Find/2(Finished) -> Unit Delay/1
  Find/1(Outputs) -> GPS Selector/2
  Through/1(Outputs) -> GPS Selector/3
  GPS Enabler/1(GPSMode) -> GPS Selector/1
  Unit Delay/1 -> GPS Enabler/1(Finished)
  GPS Selector/1 -> Outputs/1
  Through/2(Finished) -> Unit Delay1/1
  Unit Delay1/1 -> Finished/1

== system RoboBoat_SLAM_6_29/Main FSM/Termination/Output Heirarchy ==
  Desired Heading : Inport
  Sensors : Inport  Port=2
  Bus Creator{,1..2,4} (4 alike) : BusCreator  Inputs=2
  Bus Creator3 : BusCreator  Inputs=6
  C1 : Constant  Value=0
  C2 : Constant  Value=0
  C3 : Constant  Value=0
  LPTask : Constant  Value=0
  Latitude : Constant  Value=0
  Longitude : Constant  Value=0
  RPM Desired : Constant  Value=0
  Request Number : Constant  Value=10
  Outputs : Outport
  wires:
  RPM Desired/1 -> Bus Creator/1  "RPM"
  Bus Creator/1 -> Bus Creator1/1  "Control Signals"
  Bus Creator3/1 -> Bus Creator2/1  "Comms Panda"
  Request Number/1 -> Bus Creator3/1  "Request Number"
  Latitude/1 -> Bus Creator3/2  "Latitude"
  Longitude/1 -> Bus Creator3/3  "Longitude"
  C1/1 -> Bus Creator3/4  "C1"
  LPTask/1 -> Bus Creator2/2  "LIDAR Panda"
  Desired Heading/1 -> Bus Creator/2  "Desired Heading"
  Bus Creator1/1 -> Bus Creator4/1  "Outputs"
  Sensors/1 -> Bus Creator4/2  "Sensors"
  Bus Creator4/1 -> Outputs/1  "Output Signals"
  Bus Creator2/1 -> Bus Creator1/2  "Serial Outputs"
  C2/1 -> Bus Creator3/5  "C2"
  C3/1 -> Bus Creator3/6  "C3"

== system RoboBoat_SLAM_6_29/Sensors/1020 Comms/ Raspberry Pi LCM (Acoustic) ==
  LCM Input : Inport
  ASCII Decode 6 : xpcseriallib/ASCII Decode   format=Deploy:%1u, Elapsed:%g, Bearing1:%g Bearing2:%g \r\n  nvars=4  vartypes={}
  Bus Creator : BusCreator  Inputs=2
  Bus Creator1 : BusCreator  Inputs=3
  FIFO ASCII read 1 : xpcseriallib/FIFO ASCII read   header={'Deploy:'}  term=[13 10]  hold=Zero output if no new data  enable=off  maxsize=1024  outputtype=8 bit uint null terminated  sampletime=-1
  LCM Output : Outport
  wires:
  LCM Input/1 -> FIFO ASCII read 1/1
  FIFO ASCII read 1/1 -> ASCII Decode 6/1
  ASCII Decode 6/3 -> Bus Creator/1  "Horizontal Bearing"
  ASCII Decode 6/4 -> Bus Creator/2  "Vertical Bearing"
  Bus Creator/1 -> Bus Creator1/3  "Bearings"
  ASCII Decode 6/2 -> Bus Creator1/2  "Elapsed Time"
  ASCII Decode 6/1 -> Bus Creator1/1  "Deployed"
  Bus Creator1/1 -> LCM Output/1  "Acoustic Message"

== system RoboBoat_SLAM_6_29/Sensors/1020 Comms/ Raspberry Pi LCM (Navigation and Acoustics) ==
  LCM Input : Inport
  ASCII Decode 6 : xpcseriallib/ASCII Decode   format=P1:%f P2:%f P3:%f V1:%f V2:%f V3:%f E1:%f E2:%f E3:%f Pt1:%f Pt2:%f St1:%f St2:%f Start:%f Elapsed:%f RC:%d Deploy:%u, Elapsed:%g, Bearing1:%g Bearing2:%g \r\n  nvars=22  vartypes={}
  Bus Creator{,5..7} (4 alike) : BusCreator  Inputs=2
  Bus Creator{1..3,8} (4 alike) : BusCreator  Inputs=3
  Bus Creator4 : BusCreator  Inputs=9
  Data Type Conversion : DataTypeConversion  OutDataTypeStr=double
  FIFO ASCII read 1 : xpcseriallib/FIFO ASCII read   header={'P1:'}  term=[13 10]  hold=Zero output if no new data  enable=off  maxsize=2048  outputtype=8 bit uint null terminated  sampletime=-1
  Navigation LCM : Outport
  Acoustic LCM : Outport  Port=2
  wires:
  LCM Input/1 -> FIFO ASCII read 1/1
  FIFO ASCII read 1/1 -> ASCII Decode 6/1
  Bus Creator4/1 -> Navigation LCM/1  "Navigation Message"
  ASCII Decode 6/1 -> Bus Creator1/1  "X"
  ASCII Decode 6/2 -> Bus Creator1/2  "Y"
  ASCII Decode 6/3 -> Bus Creator1/3  "Psi"
  Bus Creator1/1 -> Bus Creator4/1  "Pose"
  ASCII Decode 6/4 -> Bus Creator2/1  "u"
  ASCII Decode 6/5 -> Bus Creator2/2  "v"
  Bus Creator2/1 -> Bus Creator4/2  "Velocity"
  ASCII Decode 6/7 -> Bus Creator3/1  "Roll"
  ASCII Decode 6/8 -> Bus Creator3/2  "Pitch"
  ASCII Decode 6/9 -> Bus Creator3/3  "Yaw"
  Bus Creator3/1 -> Bus Creator4/3  "Euler"
  Bus Creator5/1 -> Bus Creator4/5  "Port"
  Bus Creator6/1 -> Bus Creator4/6  "Stbd"
  ASCII Decode 6/14 -> Bus Creator6/1  "StThrust"
  ASCII Decode 6/15 -> Bus Creator6/2  "StAzimuth"
  ASCII Decode 6/12 -> Bus Creator5/1  "PtThrust"
  ASCII Decode 6/13 -> Bus Creator5/2  "PtAzimuth"
  ASCII Decode 6/16 -> Bus Creator4/7  "Start"
  ASCII Decode 6/17 -> Bus Creator4/8  "Elapsed"
  ASCII Decode 6/18 -> Data Type Conversion/1  "On/Off/RC/Auto"
  Data Type Conversion/1 -> Bus Creator4/9  "On/Off/RC/Auto"
  ASCII Decode 6/6 -> Bus Creator2/3  "r"
  ASCII Decode 6/10 -> Bus Creator7/1  "Lat"
  ASCII Decode 6/11 -> Bus Creator7/2  "Long"
  Bus Creator7/1 -> Bus Creator4/4  "GPS (LLA)"
  ASCII Decode 6/21 -> Bus Creator/1  "Horizontal Bearing"
  ASCII Decode 6/22 -> Bus Creator/2  "Vertical Bearing"
  Bus Creator/1 -> Bus Creator8/3  "Bearings"
  ASCII Decode 6/20 -> Bus Creator8/2  "Elapsed Time"
  ASCII Decode 6/19 -> Bus Creator8/1  "Deployed"
  Bus Creator8/1 -> Acoustic LCM/1  "Acoustic Message"

== system RoboBoat_SLAM_6_29/Sensors/1020 Comms/ Raspberry Pi LCM (Navigation) ==
  LCM Input : Inport
  ASCII Decode 6 : xpcseriallib/ASCII Decode   format=P1:%f P2:%f P3:%f V1:%f V2:%f V3:%f E1:%f E2:%f E3:%f Lat:%f Long:%f Pt1:%f Pt2:%f St1:%f St2:%f Start:%f Elapsed:%f RC:%d Deploy:%u Elapsed:%f Bearing1:%f Bearing2:%f Range:%f X_Pos:%f Y_Pos:%f \r\n  nvars=25  vartypes={}
  Bus Creator1 : BusCreator  Inputs=3
  Bus Creator2 : BusCreator  Inputs=3
  Bus Creator3 : BusCreator  Inputs=3
  Bus Creator4 : BusCreator  Inputs=9
  Bus Creator5 : BusCreator  Inputs=2
  Bus Creator6 : BusCreator  Inputs=2
  Bus Creator7 : BusCreator  Inputs=2
  Bus Creator8 : BusCreator  Inputs=7
  Data Type Conversion : DataTypeConversion  OutDataTypeStr=double
  FIFO ASCII read 1 : xpcseriallib/FIFO ASCII read   header={'P1:'}  term=[13 10]  hold=Zero output if no new data  enable=off  maxsize=2000  outputtype=8 bit uint null terminated  sampletime=-1
  LCM Output : Outport
  Acou LCM : Outport  Port=2
  wires:
  LCM Input/1 -> FIFO ASCII read 1/1
  FIFO ASCII read 1/1 -> ASCII Decode 6/1
  Bus Creator4/1 -> LCM Output/1  "Navigation Message"
  ASCII Decode 6/1 -> Bus Creator1/1  "X"
  ASCII Decode 6/2 -> Bus Creator1/2  "Y"
  ASCII Decode 6/3 -> Bus Creator1/3  "Psi"
  Bus Creator1/1 -> Bus Creator4/1  "Pose"
  ASCII Decode 6/4 -> Bus Creator2/1  "u"
  ASCII Decode 6/5 -> Bus Creator2/2  "v"
  Bus Creator2/1 -> Bus Creator4/2  "Velocity"
  ASCII Decode 6/7 -> Bus Creator3/1  "Roll"
  ASCII Decode 6/8 -> Bus Creator3/2  "Pitch"
  ASCII Decode 6/9 -> Bus Creator3/3  "Yaw"
  Bus Creator3/1 -> Bus Creator4/3  "Euler"
  Bus Creator5/1 -> Bus Creator4/5  "Port"
  Bus Creator6/1 -> Bus Creator4/6  "Stbd"
  ASCII Decode 6/14 -> Bus Creator6/1  "StThrust"
  ASCII Decode 6/15 -> Bus Creator6/2  "StAzimuth"
  ASCII Decode 6/12 -> Bus Creator5/1  "PtThrust"
  ASCII Decode 6/13 -> Bus Creator5/2  "PtAzimuth"
  ASCII Decode 6/16 -> Bus Creator4/7  "Start"
  ASCII Decode 6/17 -> Bus Creator4/8  "Elapsed"
  ASCII Decode 6/18 -> Data Type Conversion/1  "On/Off/RC/Auto"
  Data Type Conversion/1 -> Bus Creator4/9  "On/Off/RC/Auto"
  ASCII Decode 6/6 -> Bus Creator2/3  "r"
  ASCII Decode 6/10 -> Bus Creator7/1  "Lat"
  ASCII Decode 6/11 -> Bus Creator7/2  "Long"
  Bus Creator7/1 -> Bus Creator4/4  "GPS (LLA)"
  ASCII Decode 6/19 -> Bus Creator8/1  "Deployed"
  ASCII Decode 6/20 -> Bus Creator8/2  "Elapsed Time"
  ASCII Decode 6/21 -> Bus Creator8/3  "Horizontal Bearing"
  ASCII Decode 6/22 -> Bus Creator8/4  "Vertical Bearing"
  ASCII Decode 6/23 -> Bus Creator8/5  "Range"
  ASCII Decode 6/24 -> Bus Creator8/6  "X Pos"
  ASCII Decode 6/25 -> Bus Creator8/7  "Y Pos"
  Bus Creator8/1 -> Acou LCM/1

== system RoboBoat_SLAM_6_29/Sensors/1020 Comms/Acoustic LCM ==
  LCM Input : Inport
  Bus Creator : BusCreator  Inputs=2
  Bus Creator1 : BusCreator
  Bus Creator2 : BusCreator  Inputs=3
  Bus Selector : BusSelector  OutputSignals=Deployed,Elapsed Time,Horizontal Bearing,Vertical Bearing,Range,X Pos,Y Pos
  LCM Output : Outport
  wires:
  Bus Selector/3 -> Bus Creator/1  "<Horizontal Bearing>"
  Bus Selector/4 -> Bus Creator/2  "<Vertical Bearing>"
  Bus Creator/1 -> Bus Creator1/3  "Bearings"
  Bus Selector/2 -> Bus Creator1/2  "<Elapsed Time>"
  Bus Selector/1 -> Bus Creator1/1  "<Deployed>"
  Bus Creator1/1 -> LCM Output/1  "Acoustic Message"
  LCM Input/1 -> Bus Selector/1
  Bus Selector/5 -> Bus Creator2/1  "<Range>"
  Bus Selector/6 -> Bus Creator2/2  "<X Pos>"
  Bus Selector/7 -> Bus Creator2/3  "<Y Pos>"
  Bus Creator2/1 -> Bus Creator1/4  "Pose Estimate"

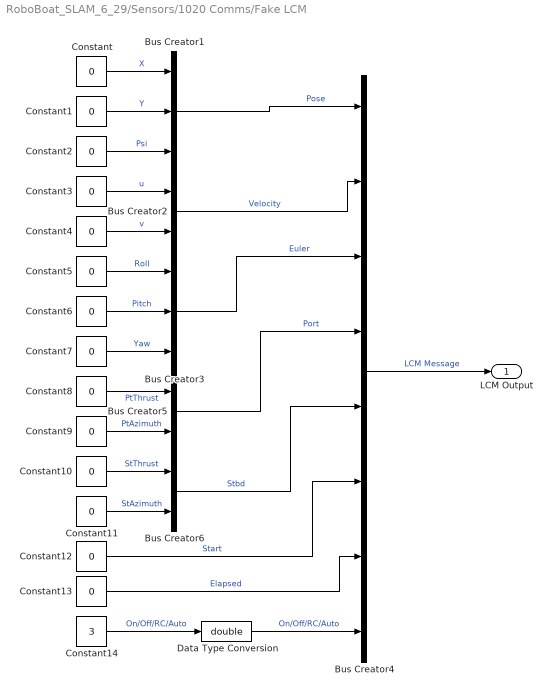
== system RoboBoat_SLAM_6_29/Sensors/1020 Comms/Fake LCM ==
  Bus Creator1 : BusCreator  Inputs=3
  Bus Creator2 : BusCreator  Inputs=2
  Bus Creator3 : BusCreator  Inputs=3
  Bus Creator4 : BusCreator  Inputs=8
  Bus Creator5 : BusCreator  Inputs=2
  Bus Creator6 : BusCreator  Inputs=2
  Constant{,1..13} (14 alike) : Constant  Value=0
  Constant14 : Constant  Value=3
  Data Type Conversion : DataTypeConversion  OutDataTypeStr=double
  LCM Output : Outport
  wires:
  Bus Creator4/1 -> LCM Output/1  "LCM Message"
  Constant/1 -> Bus Creator1/1  "X"
  Constant1/1 -> Bus Creator1/2  "Y"
  Constant2/1 -> Bus Creator1/3  "Psi"
  Bus Creator1/1 -> Bus Creator4/1  "Pose"
  Constant3/1 -> Bus Creator2/1  "u"
  Constant4/1 -> Bus Creator2/2  "v"
  Bus Creator2/1 -> Bus Creator4/2  "Velocity"
  Constant5/1 -> Bus Creator3/1  "Roll"
  Constant6/1 -> Bus Creator3/2  "Pitch"
  Constant7/1 -> Bus Creator3/3  "Yaw"
  Bus Creator3/1 -> Bus Creator4/3  "Euler"
  Bus Creator5/1 -> Bus Creator4/4  "Port"
  Bus Creator6/1 -> Bus Creator4/5  "Stbd"
  Constant10/1 -> Bus Creator6/1  "StThrust"
  Constant11/1 -> Bus Creator6/2  "StAzimuth"
  Constant8/1 -> Bus Creator5/1  "PtThrust"
  Constant9/1 -> Bus Creator5/2  "PtAzimuth"
  Constant12/1 -> Bus Creator4/6  "Start"
  Constant13/1 -> Bus Creator4/7  "Elapsed"
  Constant14/1 -> Data Type Conversion/1  "On/Off/RC/Auto"
  Data Type Conversion/1 -> Bus Creator4/8  "On/Off/RC/Auto"

== system RoboBoat_SLAM_6_29/Sensors/1020 Comms/LIDAR Panda ==
  LIDAR Panda In : Inport
  ASCII Decode 2 : xpcseriallib/ASCII Decode   format=A:%d B:%d C:%d E:%d F:%d G:%d H:%d I:%d J:%d K:%d L:%d M:%d N:%d O:%d P:%d Q:%d R:%d S:%d T:%d U:%d V:%d W:%d X:%d C1:%d C2:%d C3:%d C4:%d P1:%f P2:%f P3:%f P4:%f I1:%d I2:%d I3:%d I4:%d \r\n  nvars=36  vartypes={}
  Bus Creator1 : BusCreator  Inputs=2
  Bus Creator2 : BusCreator  Inputs=3
  Bus Creator3 : BusCreator  Inputs=2
  Data Type Conversion{,1..3} (4 alike) : DataTypeConversion  OutDataTypeStr=double
  "FIFO ASCII read " : xpcseriallib/FIFO ASCII read   header={'A:'}  term=[13 10]  hold=Zero output if no new data  enable=off  maxsize=1024  outputtype=8 bit uint null terminated  sampletime=-1
  Mux : Mux  Inputs=12
  Mux1 : Mux
  Mux2 : Mux  Inputs=12
  Mux3 : Mux
  Mux4 : Mux
  LIDAR Panda Out : Outport
  wires:
  LIDAR Panda In/1 -> "FIFO ASCII read "/1
  "FIFO ASCII read "/1 -> ASCII Decode 2/1
  ASCII Decode 2/3 -> Mux/3  "Distance"
  ASCII Decode 2/2 -> Mux/2  "Color ID"
  ASCII Decode 2/4 -> Mux/4  "Angle"
  ASCII Decode 2/1 -> Mux/1  "Probability"
  ASCII Decode 2/7 -> Mux/7
  ASCII Decode 2/10 -> Mux/10
  ASCII Decode 2/11 -> Mux/11
  ASCII Decode 2/6 -> Mux/6
  ASCII Decode 2/8 -> Mux/8
  ASCII Decode 2/9 -> Mux/9
  ASCII Decode 2/12 -> Mux/12
  ASCII Decode 2/5 -> Mux/5
  ASCII Decode 2/13 -> Mux2/1
  ASCII Decode 2/15 -> Mux2/3
  ASCII Decode 2/22 -> Mux2/10
  ASCII Decode 2/23 -> Mux2/11
  ASCII Decode 2/17 -> Mux2/5
  ASCII Decode 2/18 -> Mux2/6
  ASCII Decode 2/14 -> Mux2/2
  ASCII Decode 2/24 -> Mux2/12
  ASCII Decode 2/20 -> Mux2/8
  ASCII Decode 2/19 -> Mux2/7
  ASCII Decode 2/21 -> Mux2/9
  ASCII Decode 2/16 -> Mux2/4
  ASCII Decode 2/25 -> Mux1/1
  ASCII Decode 2/28 -> Mux1/4
  ASCII Decode 2/26 -> Mux1/2
  ASCII Decode 2/27 -> Mux1/3
  ASCII Decode 2/30 -> Mux3/2
  ASCII Decode 2/31 -> Mux3/3
  ASCII Decode 2/32 -> Mux3/4
  ASCII Decode 2/29 -> Mux3/1
  ASCII Decode 2/36 -> Mux4/4
  ASCII Decode 2/34 -> Mux4/2
  ASCII Decode 2/35 -> Mux4/3
  ASCII Decode 2/33 -> Mux4/1
  Mux/1 -> Data Type Conversion/1  "Distances"
  Mux2/1 -> Data Type Conversion1/1  "Angles"
  Mux1/1 -> Data Type Conversion2/1  "Color"
  Mux3/1 -> Bus Creator2/2  "Probability"
  Mux4/1 -> Data Type Conversion3/1  "idx"
  Bus Creator1/1 -> Bus Creator3/1  "Landmarks"
  Bus Creator2/1 -> Bus Creator3/2  "Color data"
  Bus Creator3/1 -> LIDAR Panda Out/1
  Data Type Conversion/1 -> Bus Creator1/1  "Distances"
  Data Type Conversion1/1 -> Bus Creator1/2  "Angles"
  Data Type Conversion2/1 -> Bus Creator2/1  "Color"
  Data Type Conversion3/1 -> Bus Creator2/3  "Color"

== system RoboBoat_SLAM_6_29/Sensors/1020 Comms/Subsystem ==
  Bus Creator : BusCreator  Inputs=3
  Bus Creator1 : BusCreator  Inputs=2
  Bus Creator2 : BusCreator  Inputs=2
  Constant : Constant  Value=zeros(12,1)
  Constant1 : Constant  Value=zeros(12,1)
  Constant2 : Constant  Value=zeros(4,1)
  Constant3 : Constant  Value=zeros(4,1)
  Constant4 : Constant  Value=zeros(4,1)
  Fake Panda : Outport
  wires:
  Constant/1 -> Bus Creator1/1  "Distances"
  Constant1/1 -> Bus Creator1/2  "Angles"
  Constant2/1 -> Bus Creator/1  "Color"
  Constant3/1 -> Bus Creator/2  "Probability"
  Constant4/1 -> Bus Creator/3  "idx"
  Bus Creator1/1 -> Bus Creator2/1  "Landmarks"
  Bus Creator/1 -> Bus Creator2/2  "Color data"
  Bus Creator2/1 -> Fake Panda/1  "Lidar Data Input"
